simulink model "signal_tranmission"  (R2024b)
settings: Solver=ode45  StartTime=0.0  StopTime=10  FixedStep=0.000125  RelTol=1e-3
libraries: dspfdesign x500, commchan3 x1
(part 2 of 7)

== system signal_tranmission/SSB Demod ==
  Input Signal : Inport
  Analog Filter Design1 : dspfdesign/Analog Filter Design  method=Butterworth  filttype=Lowpass  N=4  Wlo=5*2*pi  Whi=102*2*pi  Rp=2  Rs=40
  Balanced Modulator1 : Subsystem
  carrier signal : Sin  Frequency=100*2*pi  SampleTime=0
  Out1 : Outport
  wires:
  Analog Filter Design1/1 -> Out1/1
  Balanced Modulator1/1(DSBSC) -> Analog Filter Design1/1
  carrier signal/1 -> Balanced Modulator1/2(Carrier Signal)
  Input Signal/1 -> Balanced Modulator1/1(Input Signal)

== system signal_tranmission/SSB Demod1 ==
  Input Signal : Inport
  Analog Filter Design1 : dspfdesign/Analog Filter Design  method=Butterworth  filttype=Lowpass  N=4  Wlo=5*2*pi  Whi=102*2*pi  Rp=2  Rs=40
  Balanced Modulator1 : Subsystem
  carrier signal : Sin  Frequency=104*2*pi  SampleTime=0
  Out1 : Outport
  wires:
  Analog Filter Design1/1 -> Out1/1
  Balanced Modulator1/1(DSBSC) -> Analog Filter Design1/1
  carrier signal/1 -> Balanced Modulator1/2(Carrier Signal)
  Input Signal/1 -> Balanced Modulator1/1(Input Signal)

== system signal_tranmission/SSB Demod10 ==
  Input Signal : Inport
  Analog Filter Design1 : dspfdesign/Analog Filter Design  method=Butterworth  filttype=Lowpass  N=4  Wlo=5*2*pi  Whi=102*2*pi  Rp=2  Rs=40
  Balanced Modulator1 : Subsystem
  carrier signal : Sin  Frequency=140*2*pi  SampleTime=0
  Out1 : Outport
  wires:
  Analog Filter Design1/1 -> Out1/1
  Balanced Modulator1/1(DSBSC) -> Analog Filter Design1/1
  carrier signal/1 -> Balanced Modulator1/2(Carrier Signal)
  Input Signal/1 -> Balanced Modulator1/1(Input Signal)

== system signal_tranmission/SSB Demod11 ==
  Input Signal : Inport
  Analog Filter Design1 : dspfdesign/Analog Filter Design  method=Butterworth  filttype=Lowpass  N=4  Wlo=5*2*pi  Whi=102*2*pi  Rp=2  Rs=40
  Balanced Modulator1 : Subsystem
  carrier signal : Sin  Frequency=144*2*pi  SampleTime=0
  Out1 : Outport
  wires:
  Analog Filter Design1/1 -> Out1/1
  Balanced Modulator1/1(DSBSC) -> Analog Filter Design1/1
  carrier signal/1 -> Balanced Modulator1/2(Carrier Signal)
  Input Signal/1 -> Balanced Modulator1/1(Input Signal)

== system signal_tranmission/SSB Demod12 ==
  Input Signal : Inport
  Analog Filter Design1 : dspfdesign/Analog Filter Design  method=Butterworth  filttype=Lowpass  N=4  Wlo=5*2*pi  Whi=102*2*pi  Rp=2  Rs=40
  Balanced Modulator1 : Subsystem
  carrier signal : Sin  Frequency=148*2*pi  SampleTime=0
  Out1 : Outport
  wires:
  Analog Filter Design1/1 -> Out1/1
  Balanced Modulator1/1(DSBSC) -> Analog Filter Design1/1
  carrier signal/1 -> Balanced Modulator1/2(Carrier Signal)
  Input Signal/1 -> Balanced Modulator1/1(Input Signal)

== system signal_tranmission/SSB Demod13 ==
  Input Signal : Inport
  Analog Filter Design1 : dspfdesign/Analog Filter Design  method=Butterworth  filttype=Lowpass  N=4  Wlo=5*2*pi  Whi=102*2*pi  Rp=2  Rs=40
  Balanced Modulator1 : Subsystem
  carrier signal : Sin  Frequency=152*2*pi  SampleTime=0
  Out1 : Outport
  wires:
  Analog Filter Design1/1 -> Out1/1
  Balanced Modulator1/1(DSBSC) -> Analog Filter Design1/1
  carrier signal/1 -> Balanced Modulator1/2(Carrier Signal)
  Input Signal/1 -> Balanced Modulator1/1(Input Signal)

== system signal_tranmission/SSB Demod14 ==
  Input Signal : Inport
  Analog Filter Design1 : dspfdesign/Analog Filter Design  method=Butterworth  filttype=Lowpass  N=4  Wlo=5*2*pi  Whi=102*2*pi  Rp=2  Rs=40
  Balanced Modulator1 : Subsystem
  carrier signal : Sin  Frequency=156*2*pi  SampleTime=0
  Out1 : Outport
  wires:
  Analog Filter Design1/1 -> Out1/1
  Balanced Modulator1/1(DSBSC) -> Analog Filter Design1/1
  carrier signal/1 -> Balanced Modulator1/2(Carrier Signal)
  Input Signal/1 -> Balanced Modulator1/1(Input Signal)

== system signal_tranmission/SSB Demod15 ==
  Input Signal : Inport
  Analog Filter Design1 : dspfdesign/Analog Filter Design  method=Butterworth  filttype=Lowpass  N=4  Wlo=5*2*pi  Whi=102*2*pi  Rp=2  Rs=40
  Balanced Modulator1 : Subsystem
  carrier signal : Sin  Frequency=160*2*pi  SampleTime=0
  Out1 : Outport
  wires:
  Analog Filter Design1/1 -> Out1/1
  Balanced Modulator1/1(DSBSC) -> Analog Filter Design1/1
  carrier signal/1 -> Balanced Modulator1/2(Carrier Signal)
  Input Signal/1 -> Balanced Modulator1/1(Input Signal)

== system signal_tranmission/SSB Demod16 ==
  Input Signal : Inport
  Analog Filter Design1 : dspfdesign/Analog Filter Design  method=Butterworth  filttype=Lowpass  N=4  Wlo=5*2*pi  Whi=102*2*pi  Rp=2  Rs=40
  Balanced Modulator1 : Subsystem
  carrier signal : Sin  Frequency=164*2*pi  SampleTime=0
  Out1 : Outport
  wires:
  Analog Filter Design1/1 -> Out1/1
  Balanced Modulator1/1(DSBSC) -> Analog Filter Design1/1
  carrier signal/1 -> Balanced Modulator1/2(Carrier Signal)
  Input Signal/1 -> Balanced Modulator1/1(Input Signal)

== system signal_tranmission/SSB Demod17 ==
  Input Signal : Inport
  Analog Filter Design1 : dspfdesign/Analog Filter Design  method=Butterworth  filttype=Lowpass  N=4  Wlo=5*2*pi  Whi=102*2*pi  Rp=2  Rs=40
  Balanced Modulator1 : Subsystem
  carrier signal : Sin  Frequency=168*2*pi  SampleTime=0
  Out1 : Outport
  wires:
  Analog Filter Design1/1 -> Out1/1
  Balanced Modulator1/1(DSBSC) -> Analog Filter Design1/1
  carrier signal/1 -> Balanced Modulator1/2(Carrier Signal)
  Input Signal/1 -> Balanced Modulator1/1(Input Signal)

== system signal_tranmission/SSB Demod18 ==
  Input Signal : Inport
  Analog Filter Design1 : dspfdesign/Analog Filter Design  method=Butterworth  filttype=Lowpass  N=4  Wlo=5*2*pi  Whi=102*2*pi  Rp=2  Rs=40
  Balanced Modulator1 : Subsystem
  carrier signal : Sin  Frequency=172*2*pi  SampleTime=0
  Out1 : Outport
  wires:
  Analog Filter Design1/1 -> Out1/1
  Balanced Modulator1/1(DSBSC) -> Analog Filter Design1/1
  carrier signal/1 -> Balanced Modulator1/2(Carrier Signal)
  Input Signal/1 -> Balanced Modulator1/1(Input Signal)

== system signal_tranmission/SSB Demod19 ==
  Input Signal : Inport
  Analog Filter Design1 : dspfdesign/Analog Filter Design  method=Butterworth  filttype=Lowpass  N=4  Wlo=5*2*pi  Whi=102*2*pi  Rp=2  Rs=40
  Balanced Modulator1 : Subsystem
  carrier signal : Sin  Frequency=176*2*pi  SampleTime=0
  Out1 : Outport
  wires:
  Analog Filter Design1/1 -> Out1/1
  Balanced Modulator1/1(DSBSC) -> Analog Filter Design1/1
  carrier signal/1 -> Balanced Modulator1/2(Carrier Signal)
  Input Signal/1 -> Balanced Modulator1/1(Input Signal)

== system signal_tranmission/SSB Demod2 ==
  Input Signal : Inport
  Analog Filter Design1 : dspfdesign/Analog Filter Design  method=Butterworth  filttype=Lowpass  N=4  Wlo=5*2*pi  Whi=102*2*pi  Rp=2  Rs=40
  Balanced Modulator1 : Subsystem
  carrier signal : Sin  Frequency=108*2*pi  SampleTime=0
  Out1 : Outport
  wires:
  Analog Filter Design1/1 -> Out1/1
  Balanced Modulator1/1(DSBSC) -> Analog Filter Design1/1
  carrier signal/1 -> Balanced Modulator1/2(Carrier Signal)
  Input Signal/1 -> Balanced Modulator1/1(Input Signal)

== system signal_tranmission/SSB Demod20 ==
  Input Signal : Inport
  Analog Filter Design1 : dspfdesign/Analog Filter Design  method=Butterworth  filttype=Lowpass  N=4  Wlo=5*2*pi  Whi=102*2*pi  Rp=2  Rs=40
  Balanced Modulator1 : Subsystem
  carrier signal : Sin  Frequency=180*2*pi  SampleTime=0
  Out1 : Outport
  wires:
  Analog Filter Design1/1 -> Out1/1
  Balanced Modulator1/1(DSBSC) -> Analog Filter Design1/1
  carrier signal/1 -> Balanced Modulator1/2(Carrier Signal)
  Input Signal/1 -> Balanced Modulator1/1(Input Signal)

== system signal_tranmission/SSB Demod21 ==
  Input Signal : Inport
  Analog Filter Design1 : dspfdesign/Analog Filter Design  method=Butterworth  filttype=Lowpass  N=4  Wlo=5*2*pi  Whi=102*2*pi  Rp=2  Rs=40
  Balanced Modulator1 : Subsystem
  carrier signal : Sin  Frequency=184*2*pi  SampleTime=0
  Out1 : Outport
  wires:
  Analog Filter Design1/1 -> Out1/1
  Balanced Modulator1/1(DSBSC) -> Analog Filter Design1/1
  carrier signal/1 -> Balanced Modulator1/2(Carrier Signal)
  Input Signal/1 -> Balanced Modulator1/1(Input Signal)

== system signal_tranmission/SSB Demod22 ==
  Input Signal : Inport
  Analog Filter Design1 : dspfdesign/Analog Filter Design  method=Butterworth  filttype=Lowpass  N=4  Wlo=5*2*pi  Whi=102*2*pi  Rp=2  Rs=40
  Balanced Modulator1 : Subsystem
  carrier signal : Sin  Frequency=188*2*pi  SampleTime=0
  Out1 : Outport
  wires:
  Analog Filter Design1/1 -> Out1/1
  Balanced Modulator1/1(DSBSC) -> Analog Filter Design1/1
  carrier signal/1 -> Balanced Modulator1/2(Carrier Signal)
  Input Signal/1 -> Balanced Modulator1/1(Input Signal)

== system signal_tranmission/SSB Demod23 ==
  Input Signal : Inport
  Analog Filter Design1 : dspfdesign/Analog Filter Design  method=Butterworth  filttype=Lowpass  N=4  Wlo=5*2*pi  Whi=102*2*pi  Rp=2  Rs=40
  Balanced Modulator1 : Subsystem
  carrier signal : Sin  Frequency=192*2*pi  SampleTime=0
  Out1 : Outport
  wires:
  Analog Filter Design1/1 -> Out1/1
  Balanced Modulator1/1(DSBSC) -> Analog Filter Design1/1
  carrier signal/1 -> Balanced Modulator1/2(Carrier Signal)
  Input Signal/1 -> Balanced Modulator1/1(Input Signal)

== system signal_tranmission/SSB Demod24 ==
  Input Signal : Inport
  Analog Filter Design1 : dspfdesign/Analog Filter Design  method=Butterworth  filttype=Lowpass  N=4  Wlo=5*2*pi  Whi=102*2*pi  Rp=2  Rs=40
  Balanced Modulator1 : Subsystem
  carrier signal : Sin  Frequency=196*2*pi  SampleTime=0
  Out1 : Outport
  wires:
  Analog Filter Design1/1 -> Out1/1
  Balanced Modulator1/1(DSBSC) -> Analog Filter Design1/1
  carrier signal/1 -> Balanced Modulator1/2(Carrier Signal)
  Input Signal/1 -> Balanced Modulator1/1(Input Signal)

== system signal_tranmission/SSB Demod25 ==
  Input Signal : Inport
  Analog Filter Design1 : dspfdesign/Analog Filter Design  method=Butterworth  filttype=Lowpass  N=4  Wlo=5*2*pi  Whi=102*2*pi  Rp=2  Rs=40
  Balanced Modulator1 : Subsystem
  carrier signal : Sin  Frequency=200*2*pi  SampleTime=0
  Out1 : Outport
  wires:
  Analog Filter Design1/1 -> Out1/1
  Balanced Modulator1/1(DSBSC) -> Analog Filter Design1/1
  carrier signal/1 -> Balanced Modulator1/2(Carrier Signal)
  Input Signal/1 -> Balanced Modulator1/1(Input Signal)

== system signal_tranmission/SSB Demod26 ==
  Input Signal : Inport
  Analog Filter Design1 : dspfdesign/Analog Filter Design  method=Butterworth  filttype=Lowpass  N=4  Wlo=5*2*pi  Whi=102*2*pi  Rp=2  Rs=40
  Balanced Modulator1 : Subsystem
  carrier signal : Sin  Frequency=204*2*pi  SampleTime=0
  Out1 : Outport
  wires:
  Analog Filter Design1/1 -> Out1/1
  Balanced Modulator1/1(DSBSC) -> Analog Filter Design1/1
  carrier signal/1 -> Balanced Modulator1/2(Carrier Signal)
  Input Signal/1 -> Balanced Modulator1/1(Input Signal)

== system signal_tranmission/SSB Demod27 ==
  Input Signal : Inport
  Analog Filter Design1 : dspfdesign/Analog Filter Design  method=Butterworth  filttype=Lowpass  N=4  Wlo=5*2*pi  Whi=102*2*pi  Rp=2  Rs=40
  Balanced Modulator1 : Subsystem
  carrier signal : Sin  Frequency=208*2*pi  SampleTime=0
  Out1 : Outport
  wires:
  Analog Filter Design1/1 -> Out1/1
  Balanced Modulator1/1(DSBSC) -> Analog Filter Design1/1
  carrier signal/1 -> Balanced Modulator1/2(Carrier Signal)
  Input Signal/1 -> Balanced Modulator1/1(Input Signal)

== system signal_tranmission/SSB Demod28 ==
  Input Signal : Inport
  Analog Filter Design1 : dspfdesign/Analog Filter Design  method=Butterworth  filttype=Lowpass  N=4  Wlo=5*2*pi  Whi=102*2*pi  Rp=2  Rs=40
  Balanced Modulator1 : Subsystem
  carrier signal : Sin  Frequency=212*2*pi  SampleTime=0
  Out1 : Outport
  wires:
  Analog Filter Design1/1 -> Out1/1
  Balanced Modulator1/1(DSBSC) -> Analog Filter Design1/1
  carrier signal/1 -> Balanced Modulator1/2(Carrier Signal)
  Input Signal/1 -> Balanced Modulator1/1(Input Signal)

== system signal_tranmission/SSB Demod29 ==
  Input Signal : Inport
  Analog Filter Design1 : dspfdesign/Analog Filter Design  method=Butterworth  filttype=Lowpass  N=4  Wlo=5*2*pi  Whi=102*2*pi  Rp=2  Rs=40
  Balanced Modulator1 : Subsystem
  carrier signal : Sin  Frequency=216*2*pi  SampleTime=0
  Out1 : Outport
  wires:
  Analog Filter Design1/1 -> Out1/1
  Balanced Modulator1/1(DSBSC) -> Analog Filter Design1/1
  carrier signal/1 -> Balanced Modulator1/2(Carrier Signal)
  Input Signal/1 -> Balanced Modulator1/1(Input Signal)

== system signal_tranmission/SSB Demod3 ==
  Input Signal : Inport
  Analog Filter Design1 : dspfdesign/Analog Filter Design  method=Butterworth  filttype=Lowpass  N=4  Wlo=5*2*pi  Whi=102*2*pi  Rp=2  Rs=40
  Balanced Modulator1 : Subsystem
  carrier signal : Sin  Frequency=112*2*pi  SampleTime=0
  Out1 : Outport
  wires:
  Analog Filter Design1/1 -> Out1/1
  Balanced Modulator1/1(DSBSC) -> Analog Filter Design1/1
  carrier signal/1 -> Balanced Modulator1/2(Carrier Signal)
  Input Signal/1 -> Balanced Modulator1/1(Input Signal)

== system signal_tranmission/SSB Demod30 ==
  Input Signal : Inport
  Analog Filter Design1 : dspfdesign/Analog Filter Design  method=Butterworth  filttype=Lowpass  N=4  Wlo=5*2*pi  Whi=102*2*pi  Rp=2  Rs=40
  Balanced Modulator1 : Subsystem
  carrier signal : Sin  Frequency=220*2*pi  SampleTime=0
  Out1 : Outport
  wires:
  Analog Filter Design1/1 -> Out1/1
  Balanced Modulator1/1(DSBSC) -> Analog Filter Design1/1
  carrier signal/1 -> Balanced Modulator1/2(Carrier Signal)
  Input Signal/1 -> Balanced Modulator1/1(Input Signal)

== system signal_tranmission/SSB Demod31 ==
  Input Signal : Inport
  Analog Filter Design1 : dspfdesign/Analog Filter Design  method=Butterworth  filttype=Lowpass  N=4  Wlo=5*2*pi  Whi=102*2*pi  Rp=2  Rs=40
  Balanced Modulator1 : Subsystem
  carrier signal : Sin  Frequency=224*2*pi  SampleTime=0
  Out1 : Outport
  wires:
  Analog Filter Design1/1 -> Out1/1
  Balanced Modulator1/1(DSBSC) -> Analog Filter Design1/1
  carrier signal/1 -> Balanced Modulator1/2(Carrier Signal)
  Input Signal/1 -> Balanced Modulator1/1(Input Signal)

== system signal_tranmission/SSB Demod32 ==
  Input Signal : Inport
  Analog Filter Design1 : dspfdesign/Analog Filter Design  method=Butterworth  filttype=Lowpass  N=4  Wlo=5*2*pi  Whi=102*2*pi  Rp=2  Rs=40
  Balanced Modulator1 : Subsystem
  carrier signal : Sin  Frequency=228*2*pi  SampleTime=0
  Out1 : Outport
  wires:
  Analog Filter Design1/1 -> Out1/1
  Balanced Modulator1/1(DSBSC) -> Analog Filter Design1/1
  carrier signal/1 -> Balanced Modulator1/2(Carrier Signal)
  Input Signal/1 -> Balanced Modulator1/1(Input Signal)

== system signal_tranmission/SSB Demod33 ==
  Input Signal : Inport
  Analog Filter Design1 : dspfdesign/Analog Filter Design  method=Butterworth  filttype=Lowpass  N=4  Wlo=5*2*pi  Whi=102*2*pi  Rp=2  Rs=40
  Balanced Modulator1 : Subsystem
  carrier signal : Sin  Frequency=232*2*pi  SampleTime=0
  Out1 : Outport
  wires:
  Analog Filter Design1/1 -> Out1/1
  Balanced Modulator1/1(DSBSC) -> Analog Filter Design1/1
  carrier signal/1 -> Balanced Modulator1/2(Carrier Signal)
  Input Signal/1 -> Balanced Modulator1/1(Input Signal)

== system signal_tranmission/SSB Demod34 ==
  Input Signal : Inport
  Analog Filter Design1 : dspfdesign/Analog Filter Design  method=Butterworth  filttype=Lowpass  N=4  Wlo=5*2*pi  Whi=102*2*pi  Rp=2  Rs=40
  Balanced Modulator1 : Subsystem
  carrier signal : Sin  Frequency=236*2*pi  SampleTime=0
  Out1 : Outport
  wires:
  Analog Filter Design1/1 -> Out1/1
  Balanced Modulator1/1(DSBSC) -> Analog Filter Design1/1
  carrier signal/1 -> Balanced Modulator1/2(Carrier Signal)
  Input Signal/1 -> Balanced Modulator1/1(Input Signal)

== system signal_tranmission/SSB Demod35 ==
  Input Signal : Inport
  Analog Filter Design1 : dspfdesign/Analog Filter Design  method=Butterworth  filttype=Lowpass  N=4  Wlo=5*2*pi  Whi=102*2*pi  Rp=2  Rs=40
  Balanced Modulator1 : Subsystem
  carrier signal : Sin  Frequency=240*2*pi  SampleTime=0
  Out1 : Outport
  wires:
  Analog Filter Design1/1 -> Out1/1
  Balanced Modulator1/1(DSBSC) -> Analog Filter Design1/1
  carrier signal/1 -> Balanced Modulator1/2(Carrier Signal)
  Input Signal/1 -> Balanced Modulator1/1(Input Signal)

== system signal_tranmission/SSB Demod36 ==
  Input Signal : Inport
  Analog Filter Design1 : dspfdesign/Analog Filter Design  method=Butterworth  filttype=Lowpass  N=4  Wlo=5*2*pi  Whi=102*2*pi  Rp=2  Rs=40
  Balanced Modulator1 : Subsystem
  carrier signal : Sin  Frequency=244*2*pi  SampleTime=0
  Out1 : Outport
  wires:
  Analog Filter Design1/1 -> Out1/1
  Balanced Modulator1/1(DSBSC) -> Analog Filter Design1/1
  carrier signal/1 -> Balanced Modulator1/2(Carrier Signal)
  Input Signal/1 -> Balanced Modulator1/1(Input Signal)

== system signal_tranmission/SSB Demod37 ==
  Input Signal : Inport
  Analog Filter Design1 : dspfdesign/Analog Filter Design  method=Butterworth  filttype=Lowpass  N=4  Wlo=5*2*pi  Whi=102*2*pi  Rp=2  Rs=40
  Balanced Modulator1 : Subsystem
  carrier signal : Sin  Frequency=248*2*pi  SampleTime=0
  Out1 : Outport
  wires:
  Analog Filter Design1/1 -> Out1/1
  Balanced Modulator1/1(DSBSC) -> Analog Filter Design1/1
  carrier signal/1 -> Balanced Modulator1/2(Carrier Signal)
  Input Signal/1 -> Balanced Modulator1/1(Input Signal)

== system signal_tranmission/SSB Demod38 ==
  Input Signal : Inport
  Analog Filter Design1 : dspfdesign/Analog Filter Design  method=Butterworth  filttype=Lowpass  N=4  Wlo=5*2*pi  Whi=102*2*pi  Rp=2  Rs=40
  Balanced Modulator1 : Subsystem
  carrier signal : Sin  Frequency=252*2*pi  SampleTime=0
  Out1 : Outport
  wires:
  Analog Filter Design1/1 -> Out1/1
  Balanced Modulator1/1(DSBSC) -> Analog Filter Design1/1
  carrier signal/1 -> Balanced Modulator1/2(Carrier Signal)
  Input Signal/1 -> Balanced Modulator1/1(Input Signal)

== system signal_tranmission/SSB Demod39 ==
  Input Signal : Inport
  Analog Filter Design1 : dspfdesign/Analog Filter Design  method=Butterworth  filttype=Lowpass  N=4  Wlo=5*2*pi  Whi=102*2*pi  Rp=2  Rs=40
  Balanced Modulator1 : Subsystem
  carrier signal : Sin  Frequency=256*2*pi  SampleTime=0
  Out1 : Outport
  wires:
  Analog Filter Design1/1 -> Out1/1
  Balanced Modulator1/1(DSBSC) -> Analog Filter Design1/1
  carrier signal/1 -> Balanced Modulator1/2(Carrier Signal)
  Input Signal/1 -> Balanced Modulator1/1(Input Signal)

== system signal_tranmission/SSB Demod4 ==
  Input Signal : Inport
  Analog Filter Design1 : dspfdesign/Analog Filter Design  method=Butterworth  filttype=Lowpass  N=4  Wlo=5*2*pi  Whi=102*2*pi  Rp=2  Rs=40
  Balanced Modulator1 : Subsystem
  carrier signal : Sin  Frequency=116*2*pi  SampleTime=0
  Out1 : Outport
  wires:
  Analog Filter Design1/1 -> Out1/1
  Balanced Modulator1/1(DSBSC) -> Analog Filter Design1/1
  carrier signal/1 -> Balanced Modulator1/2(Carrier Signal)
  Input Signal/1 -> Balanced Modulator1/1(Input Signal)

== system signal_tranmission/SSB Demod40 ==
  Input Signal : Inport
  Analog Filter Design1 : dspfdesign/Analog Filter Design  method=Butterworth  filttype=Lowpass  N=4  Wlo=5*2*pi  Whi=102*2*pi  Rp=2  Rs=40
  Balanced Modulator1 : Subsystem
  carrier signal : Sin  Frequency=260*2*pi  SampleTime=0
  Out1 : Outport
  wires:
  Analog Filter Design1/1 -> Out1/1
  Balanced Modulator1/1(DSBSC) -> Analog Filter Design1/1
  carrier signal/1 -> Balanced Modulator1/2(Carrier Signal)
  Input Signal/1 -> Balanced Modulator1/1(Input Signal)

== system signal_tranmission/SSB Demod41 ==
  Input Signal : Inport
  Analog Filter Design1 : dspfdesign/Analog Filter Design  method=Butterworth  filttype=Lowpass  N=4  Wlo=5*2*pi  Whi=102*2*pi  Rp=2  Rs=40
  Balanced Modulator1 : Subsystem
  carrier signal : Sin  Frequency=264*2*pi  SampleTime=0
  Out1 : Outport
  wires:
  Analog Filter Design1/1 -> Out1/1
  Balanced Modulator1/1(DSBSC) -> Analog Filter Design1/1
  carrier signal/1 -> Balanced Modulator1/2(Carrier Signal)
  Input Signal/1 -> Balanced Modulator1/1(Input Signal)

== system signal_tranmission/SSB Demod42 ==
  Input Signal : Inport
  Analog Filter Design1 : dspfdesign/Analog Filter Design  method=Butterworth  filttype=Lowpass  N=4  Wlo=5*2*pi  Whi=102*2*pi  Rp=2  Rs=40
  Balanced Modulator1 : Subsystem
  carrier signal : Sin  Frequency=268*2*pi  SampleTime=0
  Out1 : Outport
  wires:
  Analog Filter Design1/1 -> Out1/1
  Balanced Modulator1/1(DSBSC) -> Analog Filter Design1/1
  carrier signal/1 -> Balanced Modulator1/2(Carrier Signal)
  Input Signal/1 -> Balanced Modulator1/1(Input Signal)

== system signal_tranmission/SSB Demod43 ==
  Input Signal : Inport
  Analog Filter Design1 : dspfdesign/Analog Filter Design  method=Butterworth  filttype=Lowpass  N=4  Wlo=5*2*pi  Whi=102*2*pi  Rp=2  Rs=40
  Balanced Modulator1 : Subsystem
  carrier signal : Sin  Frequency=272*2*pi  SampleTime=0
  Out1 : Outport
  wires:
  Analog Filter Design1/1 -> Out1/1
  Balanced Modulator1/1(DSBSC) -> Analog Filter Design1/1
  carrier signal/1 -> Balanced Modulator1/2(Carrier Signal)
  Input Signal/1 -> Balanced Modulator1/1(Input Signal)

== system signal_tranmission/SSB Demod44 ==
  Input Signal : Inport
  Analog Filter Design1 : dspfdesign/Analog Filter Design  method=Butterworth  filttype=Lowpass  N=4  Wlo=5*2*pi  Whi=102*2*pi  Rp=2  Rs=40
  Balanced Modulator1 : Subsystem
  carrier signal : Sin  Frequency=276*2*pi  SampleTime=0
  Out1 : Outport
  wires:
  Analog Filter Design1/1 -> Out1/1
  Balanced Modulator1/1(DSBSC) -> Analog Filter Design1/1
  carrier signal/1 -> Balanced Modulator1/2(Carrier Signal)
  Input Signal/1 -> Balanced Modulator1/1(Input Signal)

== system signal_tranmission/SSB Demod45 ==
  Input Signal : Inport
  Analog Filter Design1 : dspfdesign/Analog Filter Design  method=Butterworth  filttype=Lowpass  N=4  Wlo=5*2*pi  Whi=102*2*pi  Rp=2  Rs=40
  Balanced Modulator1 : Subsystem
  carrier signal : Sin  Frequency=280*2*pi  SampleTime=0
  Out1 : Outport
  wires:
  Analog Filter Design1/1 -> Out1/1
  Balanced Modulator1/1(DSBSC) -> Analog Filter Design1/1
  carrier signal/1 -> Balanced Modulator1/2(Carrier Signal)
  Input Signal/1 -> Balanced Modulator1/1(Input Signal)

== system signal_tranmission/SSB Demod46 ==
  Input Signal : Inport
  Analog Filter Design1 : dspfdesign/Analog Filter Design  method=Butterworth  filttype=Lowpass  N=4  Wlo=5*2*pi  Whi=102*2*pi  Rp=2  Rs=40
  Balanced Modulator1 : Subsystem
  carrier signal : Sin  Frequency=284*2*pi  SampleTime=0
  Out1 : Outport
  wires:
  Analog Filter Design1/1 -> Out1/1
  Balanced Modulator1/1(DSBSC) -> Analog Filter Design1/1
  carrier signal/1 -> Balanced Modulator1/2(Carrier Signal)
  Input Signal/1 -> Balanced Modulator1/1(Input Signal)

== system signal_tranmission/SSB Demod47 ==
  Input Signal : Inport
  Analog Filter Design1 : dspfdesign/Analog Filter Design  method=Butterworth  filttype=Lowpass  N=4  Wlo=5*2*pi  Whi=102*2*pi  Rp=2  Rs=40
  Balanced Modulator1 : Subsystem
  carrier signal : Sin  Frequency=288*2*pi  SampleTime=0
  Out1 : Outport
  wires:
  Analog Filter Design1/1 -> Out1/1
  Balanced Modulator1/1(DSBSC) -> Analog Filter Design1/1
  carrier signal/1 -> Balanced Modulator1/2(Carrier Signal)
  Input Signal/1 -> Balanced Modulator1/1(Input Signal)

== system signal_tranmission/SSB Demod48 ==
  Input Signal : Inport
  Analog Filter Design1 : dspfdesign/Analog Filter Design  method=Butterworth  filttype=Lowpass  N=4  Wlo=5*2*pi  Whi=102*2*pi  Rp=2  Rs=40
  Balanced Modulator1 : Subsystem
  carrier signal : Sin  Frequency=292*2*pi  SampleTime=0
  Out1 : Outport
  wires:
  Analog Filter Design1/1 -> Out1/1
  Balanced Modulator1/1(DSBSC) -> Analog Filter Design1/1
  carrier signal/1 -> Balanced Modulator1/2(Carrier Signal)
  Input Signal/1 -> Balanced Modulator1/1(Input Signal)

== system signal_tranmission/SSB Demod49 ==
  Input Signal : Inport
  Analog Filter Design1 : dspfdesign/Analog Filter Design  method=Butterworth  filttype=Lowpass  N=4  Wlo=5*2*pi  Whi=102*2*pi  Rp=2  Rs=40
  Balanced Modulator1 : Subsystem
  carrier signal : Sin  Frequency=296*2*pi  SampleTime=0
  Out1 : Outport
  wires:
  Analog Filter Design1/1 -> Out1/1
  Balanced Modulator1/1(DSBSC) -> Analog Filter Design1/1
  carrier signal/1 -> Balanced Modulator1/2(Carrier Signal)
  Input Signal/1 -> Balanced Modulator1/1(Input Signal)

== system signal_tranmission/SSB Demod5 ==
  Input Signal : Inport
  Analog Filter Design1 : dspfdesign/Analog Filter Design  method=Butterworth  filttype=Lowpass  N=4  Wlo=5*2*pi  Whi=102*2*pi  Rp=2  Rs=40
  Balanced Modulator1 : Subsystem
  carrier signal : Sin  Frequency=120*2*pi  SampleTime=0
  Out1 : Outport
  wires:
  Analog Filter Design1/1 -> Out1/1
  Balanced Modulator1/1(DSBSC) -> Analog Filter Design1/1
  carrier signal/1 -> Balanced Modulator1/2(Carrier Signal)
  Input Signal/1 -> Balanced Modulator1/1(Input Signal)

== system signal_tranmission/SSB Demod50 ==
  Input Signal : Inport
  Analog Filter Design1 : dspfdesign/Analog Filter Design  method=Butterworth  filttype=Lowpass  N=4  Wlo=5*2*pi  Whi=102*2*pi  Rp=2  Rs=40
  Balanced Modulator1 : Subsystem
  carrier signal : Sin  Frequency=300*2*pi  SampleTime=0
  Out1 : Outport
  wires:
  Analog Filter Design1/1 -> Out1/1
  Balanced Modulator1/1(DSBSC) -> Analog Filter Design1/1
  carrier signal/1 -> Balanced Modulator1/2(Carrier Signal)
  Input Signal/1 -> Balanced Modulator1/1(Input Signal)

== system signal_tranmission/SSB Demod51 ==
  Input Signal : Inport
  Analog Filter Design1 : dspfdesign/Analog Filter Design  method=Butterworth  filttype=Lowpass  N=4  Wlo=5*2*pi  Whi=102*2*pi  Rp=2  Rs=40
  Balanced Modulator1 : Subsystem
  carrier signal : Sin  Frequency=304*2*pi  SampleTime=0
  Out1 : Outport
  wires:
  Analog Filter Design1/1 -> Out1/1
  Balanced Modulator1/1(DSBSC) -> Analog Filter Design1/1
  carrier signal/1 -> Balanced Modulator1/2(Carrier Signal)
  Input Signal/1 -> Balanced Modulator1/1(Input Signal)

== system signal_tranmission/SSB Demod52 ==
  Input Signal : Inport
  Analog Filter Design1 : dspfdesign/Analog Filter Design  method=Butterworth  filttype=Lowpass  N=4  Wlo=5*2*pi  Whi=102*2*pi  Rp=2  Rs=40
  Balanced Modulator1 : Subsystem
  carrier signal : Sin  Frequency=308*2*pi  SampleTime=0
  Out1 : Outport
  wires:
  Analog Filter Design1/1 -> Out1/1
  Balanced Modulator1/1(DSBSC) -> Analog Filter Design1/1
  carrier signal/1 -> Balanced Modulator1/2(Carrier Signal)
  Input Signal/1 -> Balanced Modulator1/1(Input Signal)

== system signal_tranmission/SSB Demod53 ==
  Input Signal : Inport
  Analog Filter Design1 : dspfdesign/Analog Filter Design  method=Butterworth  filttype=Lowpass  N=4  Wlo=5*2*pi  Whi=102*2*pi  Rp=2  Rs=40
  Balanced Modulator1 : Subsystem
  carrier signal : Sin  Frequency=312*2*pi  SampleTime=0
  Out1 : Outport
  wires:
  Analog Filter Design1/1 -> Out1/1
  Balanced Modulator1/1(DSBSC) -> Analog Filter Design1/1
  carrier signal/1 -> Balanced Modulator1/2(Carrier Signal)
  Input Signal/1 -> Balanced Modulator1/1(Input Signal)

== system signal_tranmission/SSB Demod54 ==
  Input Signal : Inport
  Analog Filter Design1 : dspfdesign/Analog Filter Design  method=Butterworth  filttype=Lowpass  N=4  Wlo=5*2*pi  Whi=102*2*pi  Rp=2  Rs=40
  Balanced Modulator1 : Subsystem
  carrier signal : Sin  Frequency=316*2*pi  SampleTime=0
  Out1 : Outport
  wires:
  Analog Filter Design1/1 -> Out1/1
  Balanced Modulator1/1(DSBSC) -> Analog Filter Design1/1
  carrier signal/1 -> Balanced Modulator1/2(Carrier Signal)
  Input Signal/1 -> Balanced Modulator1/1(Input Signal)

== system signal_tranmission/SSB Demod55 ==
  Input Signal : Inport
  Analog Filter Design1 : dspfdesign/Analog Filter Design  method=Butterworth  filttype=Lowpass  N=4  Wlo=5*2*pi  Whi=102*2*pi  Rp=2  Rs=40
  Balanced Modulator1 : Subsystem
  carrier signal : Sin  Frequency=320*2*pi  SampleTime=0
  Out1 : Outport
  wires:
  Analog Filter Design1/1 -> Out1/1
  Balanced Modulator1/1(DSBSC) -> Analog Filter Design1/1
  carrier signal/1 -> Balanced Modulator1/2(Carrier Signal)
  Input Signal/1 -> Balanced Modulator1/1(Input Signal)

== system signal_tranmission/SSB Demod56 ==
  Input Signal : Inport
  Analog Filter Design1 : dspfdesign/Analog Filter Design  method=Butterworth  filttype=Lowpass  N=4  Wlo=5*2*pi  Whi=102*2*pi  Rp=2  Rs=40
  Balanced Modulator1 : Subsystem
  carrier signal : Sin  Frequency=324*2*pi  SampleTime=0
  Out1 : Outport
  wires:
  Analog Filter Design1/1 -> Out1/1
  Balanced Modulator1/1(DSBSC) -> Analog Filter Design1/1
  carrier signal/1 -> Balanced Modulator1/2(Carrier Signal)
  Input Signal/1 -> Balanced Modulator1/1(Input Signal)

== system signal_tranmission/SSB Demod57 ==
  Input Signal : Inport
  Analog Filter Design1 : dspfdesign/Analog Filter Design  method=Butterworth  filttype=Lowpass  N=4  Wlo=5*2*pi  Whi=102*2*pi  Rp=2  Rs=40
  Balanced Modulator1 : Subsystem
  carrier signal : Sin  Frequency=328*2*pi  SampleTime=0
  Out1 : Outport
  wires:
  Analog Filter Design1/1 -> Out1/1
  Balanced Modulator1/1(DSBSC) -> Analog Filter Design1/1
  carrier signal/1 -> Balanced Modulator1/2(Carrier Signal)
  Input Signal/1 -> Balanced Modulator1/1(Input Signal)

== system signal_tranmission/SSB Demod58 ==
  Input Signal : Inport
  Analog Filter Design1 : dspfdesign/Analog Filter Design  method=Butterworth  filttype=Lowpass  N=4  Wlo=5*2*pi  Whi=102*2*pi  Rp=2  Rs=40
  Balanced Modulator1 : Subsystem
  carrier signal : Sin  Frequency=332*2*pi  SampleTime=0
  Out1 : Outport
  wires:
  Analog Filter Design1/1 -> Out1/1
  Balanced Modulator1/1(DSBSC) -> Analog Filter Design1/1
  carrier signal/1 -> Balanced Modulator1/2(Carrier Signal)
  Input Signal/1 -> Balanced Modulator1/1(Input Signal)

== system signal_tranmission/SSB Demod59 ==
  Input Signal : Inport
  Analog Filter Design1 : dspfdesign/Analog Filter Design  method=Butterworth  filttype=Lowpass  N=4  Wlo=5*2*pi  Whi=102*2*pi  Rp=2  Rs=40
  Balanced Modulator1 : Subsystem
  carrier signal : Sin  Frequency=336*2*pi  SampleTime=0
  Out1 : Outport
  wires:
  Analog Filter Design1/1 -> Out1/1
  Balanced Modulator1/1(DSBSC) -> Analog Filter Design1/1
  carrier signal/1 -> Balanced Modulator1/2(Carrier Signal)
  Input Signal/1 -> Balanced Modulator1/1(Input Signal)

== system signal_tranmission/SSB Demod6 ==
  Input Signal : Inport
  Analog Filter Design1 : dspfdesign/Analog Filter Design  method=Butterworth  filttype=Lowpass  N=4  Wlo=5*2*pi  Whi=102*2*pi  Rp=2  Rs=40
  Balanced Modulator1 : Subsystem
  carrier signal : Sin  Frequency=124*2*pi  SampleTime=0
  Out1 : Outport
  wires:
  Analog Filter Design1/1 -> Out1/1
  Balanced Modulator1/1(DSBSC) -> Analog Filter Design1/1
  carrier signal/1 -> Balanced Modulator1/2(Carrier Signal)
  Input Signal/1 -> Balanced Modulator1/1(Input Signal)

== system signal_tranmission/SSB Demod60 ==
  Input Signal : Inport
  Analog Filter Design1 : dspfdesign/Analog Filter Design  method=Butterworth  filttype=Lowpass  N=4  Wlo=5*2*pi  Whi=102*2*pi  Rp=2  Rs=40
  Balanced Modulator1 : Subsystem
  carrier signal : Sin  Frequency=340*2*pi  SampleTime=0
  Out1 : Outport
  wires:
  Analog Filter Design1/1 -> Out1/1
  Balanced Modulator1/1(DSBSC) -> Analog Filter Design1/1
  carrier signal/1 -> Balanced Modulator1/2(Carrier Signal)
  Input Signal/1 -> Balanced Modulator1/1(Input Signal)

== system signal_tranmission/SSB Demod61 ==
  Input Signal : Inport
  Analog Filter Design1 : dspfdesign/Analog Filter Design  method=Butterworth  filttype=Lowpass  N=4  Wlo=5*2*pi  Whi=102*2*pi  Rp=2  Rs=40
  Balanced Modulator1 : Subsystem
  carrier signal : Sin  Frequency=344*2*pi  SampleTime=0
  Out1 : Outport
  wires:
  Analog Filter Design1/1 -> Out1/1
  Balanced Modulator1/1(DSBSC) -> Analog Filter Design1/1
  carrier signal/1 -> Balanced Modulator1/2(Carrier Signal)
  Input Signal/1 -> Balanced Modulator1/1(Input Signal)

== system signal_tranmission/SSB Demod62 ==
  Input Signal : Inport
  Analog Filter Design1 : dspfdesign/Analog Filter Design  method=Butterworth  filttype=Lowpass  N=4  Wlo=5*2*pi  Whi=102*2*pi  Rp=2  Rs=40
  Balanced Modulator1 : Subsystem
  carrier signal : Sin  Frequency=348*2*pi  SampleTime=0
  Out1 : Outport
  wires:
  Analog Filter Design1/1 -> Out1/1
  Balanced Modulator1/1(DSBSC) -> Analog Filter Design1/1
  carrier signal/1 -> Balanced Modulator1/2(Carrier Signal)
  Input Signal/1 -> Balanced Modulator1/1(Input Signal)

== system signal_tranmission/SSB Demod63 ==
  Input Signal : Inport
  Analog Filter Design1 : dspfdesign/Analog Filter Design  method=Butterworth  filttype=Lowpass  N=4  Wlo=5*2*pi  Whi=102*2*pi  Rp=2  Rs=40
  Balanced Modulator1 : Subsystem
  carrier signal : Sin  Frequency=352*2*pi  SampleTime=0
  Out1 : Outport
  wires:
  Analog Filter Design1/1 -> Out1/1
  Balanced Modulator1/1(DSBSC) -> Analog Filter Design1/1
  carrier signal/1 -> Balanced Modulator1/2(Carrier Signal)
  Input Signal/1 -> Balanced Modulator1/1(Input Signal)

== system signal_tranmission/SSB Demod64 ==
  Input Signal : Inport
  Analog Filter Design1 : dspfdesign/Analog Filter Design  method=Butterworth  filttype=Lowpass  N=4  Wlo=5*2*pi  Whi=102*2*pi  Rp=2  Rs=40
  Balanced Modulator1 : Subsystem
  carrier signal : Sin  Frequency=356*2*pi  SampleTime=0
  Out1 : Outport
  wires:
  Analog Filter Design1/1 -> Out1/1
  Balanced Modulator1/1(DSBSC) -> Analog Filter Design1/1
  carrier signal/1 -> Balanced Modulator1/2(Carrier Signal)
  Input Signal/1 -> Balanced Modulator1/1(Input Signal)

== system signal_tranmission/SSB Demod65 ==
  Input Signal : Inport
  Analog Filter Design1 : dspfdesign/Analog Filter Design  method=Butterworth  filttype=Lowpass  N=4  Wlo=5*2*pi  Whi=102*2*pi  Rp=2  Rs=40
  Balanced Modulator1 : Subsystem
  carrier signal : Sin  Frequency=360*2*pi  SampleTime=0
  Out1 : Outport
  wires:
  Analog Filter Design1/1 -> Out1/1
  Balanced Modulator1/1(DSBSC) -> Analog Filter Design1/1
  carrier signal/1 -> Balanced Modulator1/2(Carrier Signal)
  Input Signal/1 -> Balanced Modulator1/1(Input Signal)

== system signal_tranmission/SSB Demod66 ==
  Input Signal : Inport
  Analog Filter Design1 : dspfdesign/Analog Filter Design  method=Butterworth  filttype=Lowpass  N=4  Wlo=5*2*pi  Whi=102*2*pi  Rp=2  Rs=40
  Balanced Modulator1 : Subsystem
  carrier signal : Sin  Frequency=364*2*pi  SampleTime=0
  Out1 : Outport
  wires:
  Analog Filter Design1/1 -> Out1/1
  Balanced Modulator1/1(DSBSC) -> Analog Filter Design1/1
  carrier signal/1 -> Balanced Modulator1/2(Carrier Signal)
  Input Signal/1 -> Balanced Modulator1/1(Input Signal)

== system signal_tranmission/SSB Demod67 ==
  Input Signal : Inport
  Analog Filter Design1 : dspfdesign/Analog Filter Design  method=Butterworth  filttype=Lowpass  N=4  Wlo=5*2*pi  Whi=102*2*pi  Rp=2  Rs=40
  Balanced Modulator1 : Subsystem
  carrier signal : Sin  Frequency=368*2*pi  SampleTime=0
  Out1 : Outport
  wires:
  Analog Filter Design1/1 -> Out1/1
  Balanced Modulator1/1(DSBSC) -> Analog Filter Design1/1
  carrier signal/1 -> Balanced Modulator1/2(Carrier Signal)
  Input Signal/1 -> Balanced Modulator1/1(Input Signal)

== system signal_tranmission/SSB Demod68 ==
  Input Signal : Inport
  Analog Filter Design1 : dspfdesign/Analog Filter Design  method=Butterworth  filttype=Lowpass  N=4  Wlo=5*2*pi  Whi=102*2*pi  Rp=2  Rs=40
  Balanced Modulator1 : Subsystem
  carrier signal : Sin  Frequency=372*2*pi  SampleTime=0
  Out1 : Outport
  wires:
  Analog Filter Design1/1 -> Out1/1
  Balanced Modulator1/1(DSBSC) -> Analog Filter Design1/1
  carrier signal/1 -> Balanced Modulator1/2(Carrier Signal)
  Input Signal/1 -> Balanced Modulator1/1(Input Signal)

== system signal_tranmission/SSB Demod69 ==
  Input Signal : Inport
  Analog Filter Design1 : dspfdesign/Analog Filter Design  method=Butterworth  filttype=Lowpass  N=4  Wlo=5*2*pi  Whi=102*2*pi  Rp=2  Rs=40
  Balanced Modulator1 : Subsystem
  carrier signal : Sin  Frequency=376*2*pi  SampleTime=0
  Out1 : Outport
  wires:
  Analog Filter Design1/1 -> Out1/1
  Balanced Modulator1/1(DSBSC) -> Analog Filter Design1/1
  carrier signal/1 -> Balanced Modulator1/2(Carrier Signal)
  Input Signal/1 -> Balanced Modulator1/1(Input Signal)

== system signal_tranmission/SSB Demod7 ==
  Input Signal : Inport
  Analog Filter Design1 : dspfdesign/Analog Filter Design  method=Butterworth  filttype=Lowpass  N=4  Wlo=5*2*pi  Whi=102*2*pi  Rp=2  Rs=40
  Balanced Modulator1 : Subsystem
  carrier signal : Sin  Frequency=128*2*pi  SampleTime=0
  Out1 : Outport
  wires:
  Analog Filter Design1/1 -> Out1/1
  Balanced Modulator1/1(DSBSC) -> Analog Filter Design1/1
  carrier signal/1 -> Balanced Modulator1/2(Carrier Signal)
  Input Signal/1 -> Balanced Modulator1/1(Input Signal)

== system signal_tranmission/SSB Demod70 ==
  Input Signal : Inport
  Analog Filter Design1 : dspfdesign/Analog Filter Design  method=Butterworth  filttype=Lowpass  N=4  Wlo=5*2*pi  Whi=102*2*pi  Rp=2  Rs=40
  Balanced Modulator1 : Subsystem
  carrier signal : Sin  Frequency=380*2*pi  SampleTime=0
  Out1 : Outport
  wires:
  Analog Filter Design1/1 -> Out1/1
  Balanced Modulator1/1(DSBSC) -> Analog Filter Design1/1
  carrier signal/1 -> Balanced Modulator1/2(Carrier Signal)
  Input Signal/1 -> Balanced Modulator1/1(Input Signal)

== system signal_tranmission/SSB Demod71 ==
  Input Signal : Inport
  Analog Filter Design1 : dspfdesign/Analog Filter Design  method=Butterworth  filttype=Lowpass  N=4  Wlo=5*2*pi  Whi=102*2*pi  Rp=2  Rs=40
  Balanced Modulator1 : Subsystem
  carrier signal : Sin  Frequency=384*2*pi  SampleTime=0
  Out1 : Outport
  wires:
  Analog Filter Design1/1 -> Out1/1
  Balanced Modulator1/1(DSBSC) -> Analog Filter Design1/1
  carrier signal/1 -> Balanced Modulator1/2(Carrier Signal)
  Input Signal/1 -> Balanced Modulator1/1(Input Signal)

== system signal_tranmission/SSB Demod72 ==
  Input Signal : Inport
  Analog Filter Design1 : dspfdesign/Analog Filter Design  method=Butterworth  filttype=Lowpass  N=4  Wlo=5*2*pi  Whi=102*2*pi  Rp=2  Rs=40
  Balanced Modulator1 : Subsystem
  carrier signal : Sin  Frequency=388*2*pi  SampleTime=0
  Out1 : Outport
  wires:
  Analog Filter Design1/1 -> Out1/1
  Balanced Modulator1/1(DSBSC) -> Analog Filter Design1/1
  carrier signal/1 -> Balanced Modulator1/2(Carrier Signal)
  Input Signal/1 -> Balanced Modulator1/1(Input Signal)

== system signal_tranmission/SSB Demod73 ==
  Input Signal : Inport
  Analog Filter Design1 : dspfdesign/Analog Filter Design  method=Butterworth  filttype=Lowpass  N=4  Wlo=5*2*pi  Whi=102*2*pi  Rp=2  Rs=40
  Balanced Modulator1 : Subsystem
  carrier signal : Sin  Frequency=392*2*pi  SampleTime=0
  Out1 : Outport
  wires:
  Analog Filter Design1/1 -> Out1/1
  Balanced Modulator1/1(DSBSC) -> Analog Filter Design1/1
  carrier signal/1 -> Balanced Modulator1/2(Carrier Signal)
  Input Signal/1 -> Balanced Modulator1/1(Input Signal)

== system signal_tranmission/SSB Demod74 ==
  Input Signal : Inport
  Analog Filter Design1 : dspfdesign/Analog Filter Design  method=Butterworth  filttype=Lowpass  N=4  Wlo=5*2*pi  Whi=102*2*pi  Rp=2  Rs=40
  Balanced Modulator1 : Subsystem
  carrier signal : Sin  Frequency=396*2*pi  SampleTime=0
  Out1 : Outport
  wires:
  Analog Filter Design1/1 -> Out1/1
  Balanced Modulator1/1(DSBSC) -> Analog Filter Design1/1
  carrier signal/1 -> Balanced Modulator1/2(Carrier Signal)
  Input Signal/1 -> Balanced Modulator1/1(Input Signal)

== system signal_tranmission/SSB Demod75 ==
  Input Signal : Inport
  Analog Filter Design1 : dspfdesign/Analog Filter Design  method=Butterworth  filttype=Lowpass  N=4  Wlo=5*2*pi  Whi=102*2*pi  Rp=2  Rs=40
  Balanced Modulator1 : Subsystem
  carrier signal : Sin  Frequency=400*2*pi  SampleTime=0
  Out1 : Outport
  wires:
  Analog Filter Design1/1 -> Out1/1
  Balanced Modulator1/1(DSBSC) -> Analog Filter Design1/1
  carrier signal/1 -> Balanced Modulator1/2(Carrier Signal)
  Input Signal/1 -> Balanced Modulator1/1(Input Signal)

== system signal_tranmission/SSB Demod76 ==
  Input Signal : Inport
  Analog Filter Design1 : dspfdesign/Analog Filter Design  method=Butterworth  filttype=Lowpass  N=4  Wlo=5*2*pi  Whi=102*2*pi  Rp=2  Rs=40
  Balanced Modulator1 : Subsystem
  carrier signal : Sin  Frequency=404*2*pi  SampleTime=0
  Out1 : Outport
  wires:
  Analog Filter Design1/1 -> Out1/1
  Balanced Modulator1/1(DSBSC) -> Analog Filter Design1/1
  carrier signal/1 -> Balanced Modulator1/2(Carrier Signal)
  Input Signal/1 -> Balanced Modulator1/1(Input Signal)

== system signal_tranmission/SSB Demod77 ==
  Input Signal : Inport
  Analog Filter Design1 : dspfdesign/Analog Filter Design  method=Butterworth  filttype=Lowpass  N=4  Wlo=5*2*pi  Whi=102*2*pi  Rp=2  Rs=40
  Balanced Modulator1 : Subsystem
  carrier signal : Sin  Frequency=408*2*pi  SampleTime=0
  Out1 : Outport
  wires:
  Analog Filter Design1/1 -> Out1/1
  Balanced Modulator1/1(DSBSC) -> Analog Filter Design1/1
  carrier signal/1 -> Balanced Modulator1/2(Carrier Signal)
  Input Signal/1 -> Balanced Modulator1/1(Input Signal)

== system signal_tranmission/SSB Demod78 ==
  Input Signal : Inport
  Analog Filter Design1 : dspfdesign/Analog Filter Design  method=Butterworth  filttype=Lowpass  N=4  Wlo=5*2*pi  Whi=102*2*pi  Rp=2  Rs=40
  Balanced Modulator1 : Subsystem
  carrier signal : Sin  Frequency=412*2*pi  SampleTime=0
  Out1 : Outport
  wires:
  Analog Filter Design1/1 -> Out1/1
  Balanced Modulator1/1(DSBSC) -> Analog Filter Design1/1
  carrier signal/1 -> Balanced Modulator1/2(Carrier Signal)
  Input Signal/1 -> Balanced Modulator1/1(Input Signal)

== system signal_tranmission/SSB Demod79 ==
  Input Signal : Inport
  Analog Filter Design1 : dspfdesign/Analog Filter Design  method=Butterworth  filttype=Lowpass  N=4  Wlo=5*2*pi  Whi=102*2*pi  Rp=2  Rs=40
  Balanced Modulator1 : Subsystem
  carrier signal : Sin  Frequency=416*2*pi  SampleTime=0
  Out1 : Outport
  wires:
  Analog Filter Design1/1 -> Out1/1
  Balanced Modulator1/1(DSBSC) -> Analog Filter Design1/1
  carrier signal/1 -> Balanced Modulator1/2(Carrier Signal)
  Input Signal/1 -> Balanced Modulator1/1(Input Signal)

== system signal_tranmission/SSB Demod8 ==
  Input Signal : Inport
  Analog Filter Design1 : dspfdesign/Analog Filter Design  method=Butterworth  filttype=Lowpass  N=4  Wlo=5*2*pi  Whi=102*2*pi  Rp=2  Rs=40
  Balanced Modulator1 : Subsystem
  carrier signal : Sin  Frequency=132*2*pi  SampleTime=0
  Out1 : Outport
  wires:
  Analog Filter Design1/1 -> Out1/1
  Balanced Modulator1/1(DSBSC) -> Analog Filter Design1/1
  carrier signal/1 -> Balanced Modulator1/2(Carrier Signal)
  Input Signal/1 -> Balanced Modulator1/1(Input Signal)

== system signal_tranmission/SSB Demod80 ==
  Input Signal : Inport
  Analog Filter Design1 : dspfdesign/Analog Filter Design  method=Butterworth  filttype=Lowpass  N=4  Wlo=5*2*pi  Whi=102*2*pi  Rp=2  Rs=40
  Balanced Modulator1 : Subsystem
  carrier signal : Sin  Frequency=420*2*pi  SampleTime=0
  Out1 : Outport
  wires:
  Analog Filter Design1/1 -> Out1/1
  Balanced Modulator1/1(DSBSC) -> Analog Filter Design1/1
  carrier signal/1 -> Balanced Modulator1/2(Carrier Signal)
  Input Signal/1 -> Balanced Modulator1/1(Input Signal)

== system signal_tranmission/SSB Demod81 ==
  Input Signal : Inport
  Analog Filter Design1 : dspfdesign/Analog Filter Design  method=Butterworth  filttype=Lowpass  N=4  Wlo=5*2*pi  Whi=102*2*pi  Rp=2  Rs=40
  Balanced Modulator1 : Subsystem
  carrier signal : Sin  Frequency=424*2*pi  SampleTime=0
  Out1 : Outport
  wires:
  Analog Filter Design1/1 -> Out1/1
  Balanced Modulator1/1(DSBSC) -> Analog Filter Design1/1
  carrier signal/1 -> Balanced Modulator1/2(Carrier Signal)
  Input Signal/1 -> Balanced Modulator1/1(Input Signal)

== system signal_tranmission/SSB Demod82 ==
  Input Signal : Inport
  Analog Filter Design1 : dspfdesign/Analog Filter Design  method=Butterworth  filttype=Lowpass  N=4  Wlo=5*2*pi  Whi=102*2*pi  Rp=2  Rs=40
  Balanced Modulator1 : Subsystem
  carrier signal : Sin  Frequency=428*2*pi  SampleTime=0
  Out1 : Outport
  wires:
  Analog Filter Design1/1 -> Out1/1
  Balanced Modulator1/1(DSBSC) -> Analog Filter Design1/1
  carrier signal/1 -> Balanced Modulator1/2(Carrier Signal)
  Input Signal/1 -> Balanced Modulator1/1(Input Signal)

== system signal_tranmission/SSB Demod83 ==
  Input Signal : Inport
  Analog Filter Design1 : dspfdesign/Analog Filter Design  method=Butterworth  filttype=Lowpass  N=4  Wlo=5*2*pi  Whi=102*2*pi  Rp=2  Rs=40
  Balanced Modulator1 : Subsystem
  carrier signal : Sin  Frequency=432*2*pi  SampleTime=0
  Out1 : Outport
  wires:
  Analog Filter Design1/1 -> Out1/1
  Balanced Modulator1/1(DSBSC) -> Analog Filter Design1/1
  carrier signal/1 -> Balanced Modulator1/2(Carrier Signal)
  Input Signal/1 -> Balanced Modulator1/1(Input Signal)

== system signal_tranmission/SSB Demod84 ==
  Input Signal : Inport
  Analog Filter Design1 : dspfdesign/Analog Filter Design  method=Butterworth  filttype=Lowpass  N=4  Wlo=5*2*pi  Whi=102*2*pi  Rp=2  Rs=40
  Balanced Modulator1 : Subsystem
  carrier signal : Sin  Frequency=436*2*pi  SampleTime=0
  Out1 : Outport
  wires:
  Analog Filter Design1/1 -> Out1/1
  Balanced Modulator1/1(DSBSC) -> Analog Filter Design1/1
  carrier signal/1 -> Balanced Modulator1/2(Carrier Signal)
  Input Signal/1 -> Balanced Modulator1/1(Input Signal)

== system signal_tranmission/SSB Demod85 ==
  Input Signal : Inport
  Analog Filter Design1 : dspfdesign/Analog Filter Design  method=Butterworth  filttype=Lowpass  N=4  Wlo=5*2*pi  Whi=102*2*pi  Rp=2  Rs=40
  Balanced Modulator1 : Subsystem
  carrier signal : Sin  Frequency=440*2*pi  SampleTime=0
  Out1 : Outport
  wires:
  Analog Filter Design1/1 -> Out1/1
  Balanced Modulator1/1(DSBSC) -> Analog Filter Design1/1
  carrier signal/1 -> Balanced Modulator1/2(Carrier Signal)
  Input Signal/1 -> Balanced Modulator1/1(Input Signal)

== system signal_tranmission/SSB Demod86 ==
  Input Signal : Inport
  Analog Filter Design1 : dspfdesign/Analog Filter Design  method=Butterworth  filttype=Lowpass  N=4  Wlo=5*2*pi  Whi=102*2*pi  Rp=2  Rs=40
  Balanced Modulator1 : Subsystem
  carrier signal : Sin  Frequency=444*2*pi  SampleTime=0
  Out1 : Outport
  wires:
  Analog Filter Design1/1 -> Out1/1
  Balanced Modulator1/1(DSBSC) -> Analog Filter Design1/1
  carrier signal/1 -> Balanced Modulator1/2(Carrier Signal)
  Input Signal/1 -> Balanced Modulator1/1(Input Signal)

== system signal_tranmission/SSB Demod87 ==
  Input Signal : Inport
  Analog Filter Design1 : dspfdesign/Analog Filter Design  method=Butterworth  filttype=Lowpass  N=4  Wlo=5*2*pi  Whi=102*2*pi  Rp=2  Rs=40
  Balanced Modulator1 : Subsystem
  carrier signal : Sin  Frequency=448*2*pi  SampleTime=0
  Out1 : Outport
  wires:
  Analog Filter Design1/1 -> Out1/1
  Balanced Modulator1/1(DSBSC) -> Analog Filter Design1/1
  carrier signal/1 -> Balanced Modulator1/2(Carrier Signal)
  Input Signal/1 -> Balanced Modulator1/1(Input Signal)

== system signal_tranmission/SSB Demod88 ==
  Input Signal : Inport
  Analog Filter Design1 : dspfdesign/Analog Filter Design  method=Butterworth  filttype=Lowpass  N=4  Wlo=5*2*pi  Whi=102*2*pi  Rp=2  Rs=40
  Balanced Modulator1 : Subsystem
  carrier signal : Sin  Frequency=452*2*pi  SampleTime=0
  Out1 : Outport
  wires:
  Analog Filter Design1/1 -> Out1/1
  Balanced Modulator1/1(DSBSC) -> Analog Filter Design1/1
  carrier signal/1 -> Balanced Modulator1/2(Carrier Signal)
  Input Signal/1 -> Balanced Modulator1/1(Input Signal)

== system signal_tranmission/SSB Demod89 ==
  Input Signal : Inport
  Analog Filter Design1 : dspfdesign/Analog Filter Design  method=Butterworth  filttype=Lowpass  N=4  Wlo=5*2*pi  Whi=102*2*pi  Rp=2  Rs=40
  Balanced Modulator1 : Subsystem
  carrier signal : Sin  Frequency=456*2*pi  SampleTime=0
  Out1 : Outport
  wires:
  Analog Filter Design1/1 -> Out1/1
  Balanced Modulator1/1(DSBSC) -> Analog Filter Design1/1
  carrier signal/1 -> Balanced Modulator1/2(Carrier Signal)
  Input Signal/1 -> Balanced Modulator1/1(Input Signal)

== system signal_tranmission/SSB Demod9 ==
  Input Signal : Inport
  Analog Filter Design1 : dspfdesign/Analog Filter Design  method=Butterworth  filttype=Lowpass  N=4  Wlo=5*2*pi  Whi=102*2*pi  Rp=2  Rs=40
  Balanced Modulator1 : Subsystem
  carrier signal : Sin  Frequency=136*2*pi  SampleTime=0
  Out1 : Outport
  wires:
  Analog Filter Design1/1 -> Out1/1
  Balanced Modulator1/1(DSBSC) -> Analog Filter Design1/1
  carrier signal/1 -> Balanced Modulator1/2(Carrier Signal)
  Input Signal/1 -> Balanced Modulator1/1(Input Signal)

== system signal_tranmission/SSB Demod90 ==
  Input Signal : Inport
  Analog Filter Design1 : dspfdesign/Analog Filter Design  method=Butterworth  filttype=Lowpass  N=4  Wlo=5*2*pi  Whi=102*2*pi  Rp=2  Rs=40
  Balanced Modulator1 : Subsystem
  carrier signal : Sin  Frequency=460*2*pi  SampleTime=0
  Out1 : Outport
  wires:
  Analog Filter Design1/1 -> Out1/1
  Balanced Modulator1/1(DSBSC) -> Analog Filter Design1/1
  carrier signal/1 -> Balanced Modulator1/2(Carrier Signal)
  Input Signal/1 -> Balanced Modulator1/1(Input Signal)

== system signal_tranmission/SSB Demod91 ==
  Input Signal : Inport
  Analog Filter Design1 : dspfdesign/Analog Filter Design  method=Butterworth  filttype=Lowpass  N=4  Wlo=5*2*pi  Whi=102*2*pi  Rp=2  Rs=40
  Balanced Modulator1 : Subsystem
  carrier signal : Sin  Frequency=464*2*pi  SampleTime=0
  Out1 : Outport
  wires:
  Analog Filter Design1/1 -> Out1/1
  Balanced Modulator1/1(DSBSC) -> Analog Filter Design1/1
  carrier signal/1 -> Balanced Modulator1/2(Carrier Signal)
  Input Signal/1 -> Balanced Modulator1/1(Input Signal)
